simulink model "MotorControl_With_SafetyInterlock"  (R2025a)
settings: Solver=VariableStepAuto  StartTime=0.0  StopTime=30  RelTol=1e-3
libraries: SignalEditorBlockLib x1
settings Model: Creator=Rudransh  LastModifiedBy=Rudransh

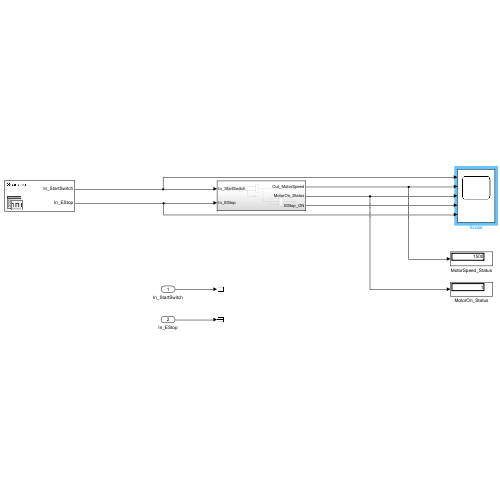
[thumbnail: Simulink's stored preview of the top-level diagram]
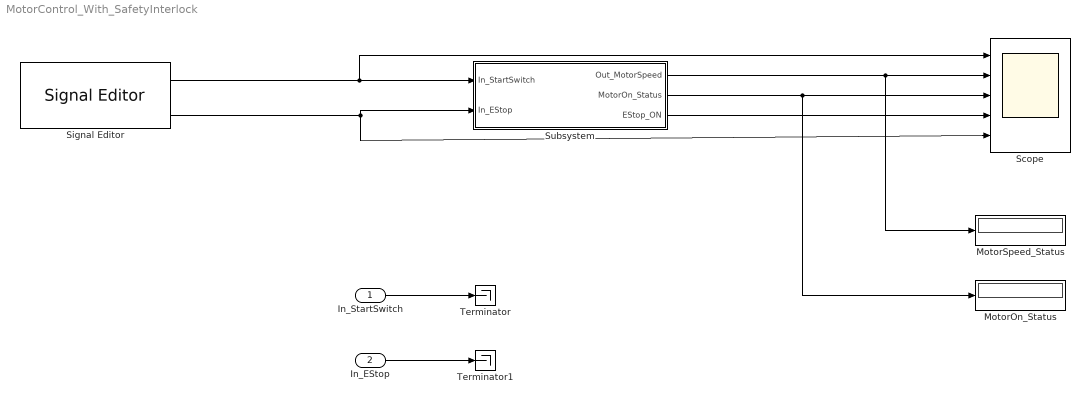
== system MotorControl_With_SafetyInterlock ==
  In_StartSwitch : Inport
  In_EStop : Inport  Port=2
  MotorOn_Status : Display
  MotorSpeed_Status : Display
  Scope : Scope  NumInputPorts=5
      settings: ActiveDisplayString=5  Title=In_EStop  ActiveDisplayYMinimum=0  ActiveDisplayYMaximum=1
  Signal Editor : SignalEditorBlockLib/Signal Editor  FileName=C:\Projects_ESD\AUTOSAR_CARSYSTEM\Motor_Control_With_Safety_Interlock\Scenario\Scenario6.mat  ActiveScenario=Scenario  ActiveSignal=In_StartSwitch  IsBus=off  OutputBusObjectStr=Bus: BusObject  SampleTime=0  ZeroCross=off  OutputAfterFinalValue=Setting to zero  Unit=inherit  PreserveSignalName=on  ApplySigPropsToAllScenarios=on  ApplySigPropsToAllSignals=off  SignalPropertySource=Dialog parameters
  Subsystem : Subsystem
  Terminator : Terminator
  Terminator1 : Terminator
  wires:
  In_EStop/1 -> Terminator1/1
  In_StartSwitch/1 -> Terminator/1
  Subsystem/1(Out_MotorSpeed) -> MotorSpeed_Status/1, Scope/2
  Subsystem/2(MotorOn_Status) -> MotorOn_Status/1, Scope/3
  Subsystem/3(EStop_ON) -> Scope/4
  Signal Editor/1 -> Scope/1, Subsystem/1(In_StartSwitch)
  Signal Editor/2 -> Scope/5, Subsystem/2(In_EStop)

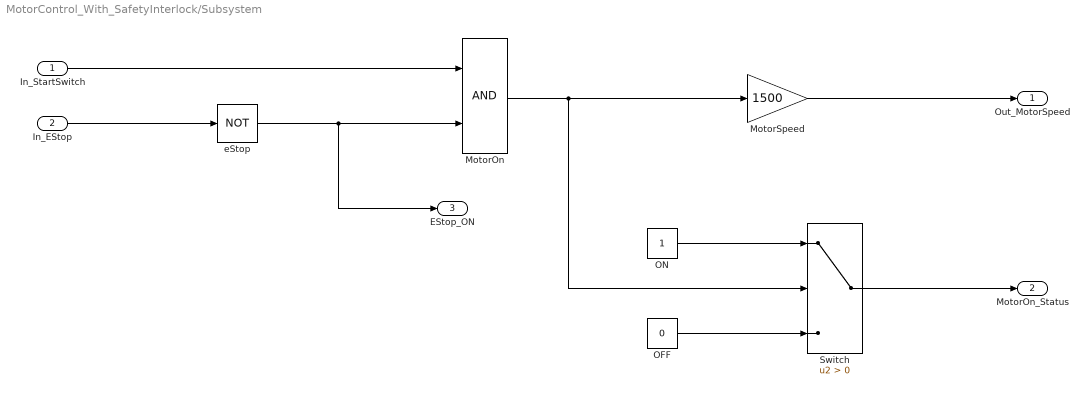
== system MotorControl_With_SafetyInterlock/Subsystem ==
  In_StartSwitch : Inport
  In_EStop : Inport  Port=2
  MotorOn : Logic  AllPortsSameDT=off  OutDataTypeStr=boolean
  MotorSpeed : Gain  Gain=1500
  OFF : Constant  Value=0
  ON : Constant
  Switch : Switch  Criteria=u2 > Threshold  SaturateOnIntegerOverflow=off  InputSameDT=off
  eStop : Logic  Operator=NOT  AllPortsSameDT=off  OutDataTypeStr=boolean
  Out_MotorSpeed : Outport
  MotorOn_Status : Outport  Port=2
  EStop_ON : Outport  Port=3
  wires:
  In_StartSwitch/1 -> MotorOn/1
  ON/1 -> Switch/1
  Switch/1 -> MotorOn_Status/1
  OFF/1 -> Switch/3
  MotorOn/1 -> Switch/2, MotorSpeed/1
  eStop/1 -> EStop_ON/1, MotorOn/2
  MotorSpeed/1 -> Out_MotorSpeed/1
  In_EStop/1 -> eStop/1
